simulink model "Langsdynamikmodell"  (R2021a)
settings: Solver=ode3  StartTime=0.0  StopTime=70  FixedStep=0.01  RelTol=1e-3
values from neighbouring files (symbols this model uses):
  A = 2    [Parameter.m]
  cw = 0.0    (= 0)    [Parameter.m]
  d = 0.63    [Parameter.m]
  m = 1500    [Parameter.m]
  p = 1.2    [Parameter.m]
undefined symbols (not defined in the file or in its folder): DiscIntNeverNeededParam
libraries: simulink x2
settings Model: Creator=ge78kon  LastModifiedBy=admin
settings SolverCC: AlgebraicLoopSolver=TrustRegion
settings DataIOCC: ReturnWorkspaceOutputs=off
settings DebuggingCC: SFMachineParentedDataDiag=warning  ArithmeticOperatorsInVariantConditions=warning
settings SFSimCC: CustomCodeUndefinedFunction=UseInterfaceOnly

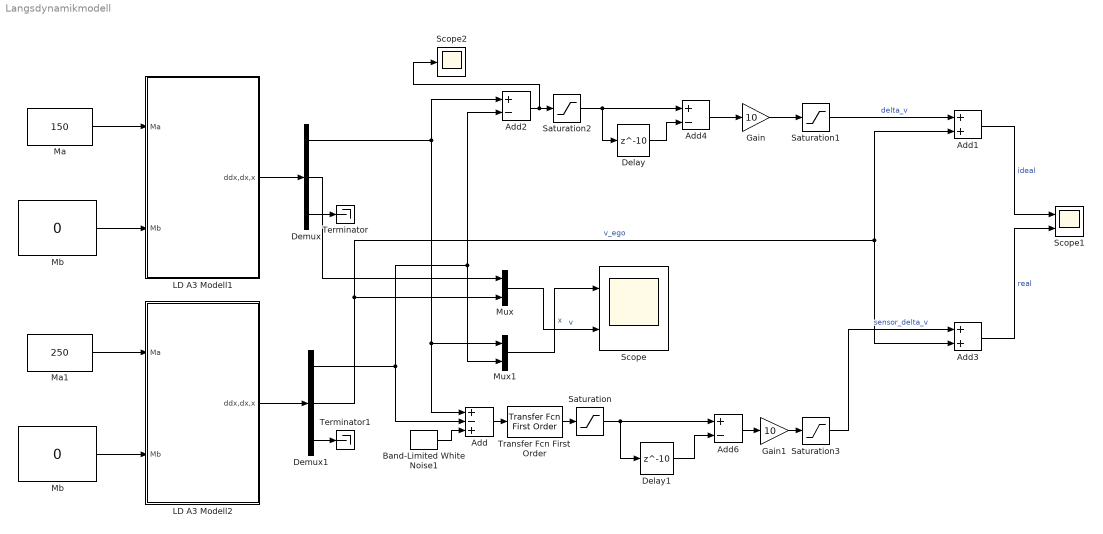
== system Langsdynamikmodell ==
  Add : Sum  Inputs=+-+
  Add1 : Sum
  Add2 : Sum  Inputs=+-
  Add3 : Sum
  Add4 : Sum  Inputs=+-
  Add6 : Sum  Inputs=+-
  Band-Limited White Noise1 : simulink/Sources/Band-Limited White Noise  Cov=[0.007]  Ts=0.01  seed=[23341]
  Delay : Delay  DelayLength=10
  Delay1 : Delay  DelayLength=10
  Demux : Demux  Outputs=3
  Demux1 : Demux  Outputs=3
  Gain : Gain  Gain=10
  Gain1 : Gain  Gain=10
  LD A3 Modell1 : Subsystem  mask{x_start=450, v_start=20}
      mask prompts: x_start "Startposition"; v_start "Startgeschwindigkeit"
  LD A3 Modell2 : Subsystem  mask{x_start=0, v_start=30}
      mask prompts: x_start "Startposition"; v_start "Startgeschwindigkeit"
  Ma : Constant  Value=150
  Ma1 : Constant  Value=250
  Mb : Constant  Value=0
  "Mb " : Constant  Value=0
  Mux : Mux  Inputs=2
  Mux1 : Mux  Inputs=2
  Saturation : Saturate  UpperLimit=200  LowerLimit=0
  Saturation1 : Saturate  UpperLimit=0  LowerLimit=-50
  Saturation2 : Saturate  UpperLimit=200  LowerLimit=0
  Saturation3 : Saturate  UpperLimit=0  LowerLimit=-50
  Scope : Scope  NumInputPorts=2
  Scope1 : Scope  NumInputPorts=2
  Scope2 : Scope
  Terminator : Terminator
  Terminator1 : Terminator
  Transfer Fcn First Order : simulink/Discrete/Transfer Fcn First Order  PoleZ=0.99  ICPrevOutput=0.0  DoSatur=off
  wires:
  Ma/1 -> LD A3 Modell1/1("Ma ")
  "Mb "/1 -> LD A3 Modell1/2("Mb ")
  LD A3 Modell1/1(ddx,dx,x) -> Demux/1
  LD A3 Modell2/1(ddx,dx,x) -> Demux1/1
  Ma1/1 -> LD A3 Modell2/1("Ma ")
  Mb/1 -> LD A3 Modell2/2("Mb ")
  Demux/3 -> Terminator/1
  Demux1/3 -> Terminator1/1
  Add6/1 -> Gain1/1
  Demux1/1 -> Add/2, Add2/2, Mux1/2
  Demux/2 -> Mux/1
  Demux1/2 -> Add1/2, Add3/2, Mux/2  "v_ego"
  Mux/1 -> Scope/2  "v"
  Mux1/1 -> Scope/1  "x"
  Add2/1 -> Scope2/1, Saturation2/1
  Add4/1 -> Gain/1
  Gain/1 -> Saturation1/1
  Band-Limited White Noise1/1 -> Add/3
  Demux/1 -> Mux1/1, Add/1, Add2/1
  Delay/1 -> Add4/2
  Delay1/1 -> Add6/2
  Saturation/1 -> Delay1/1, Add6/1
  Saturation2/1 -> Delay/1, Add4/1
  Saturation3/1 -> Add3/1  "sensor_delta_v"
  Add/1 -> Transfer Fcn First Order/1
  Gain1/1 -> Saturation3/1
  Transfer Fcn First Order/1 -> Saturation/1
  Saturation1/1 -> Add1/1  "delta_v"
  Add1/1 -> Scope1/1  "ideal"
  Add3/1 -> Scope1/2  "real"

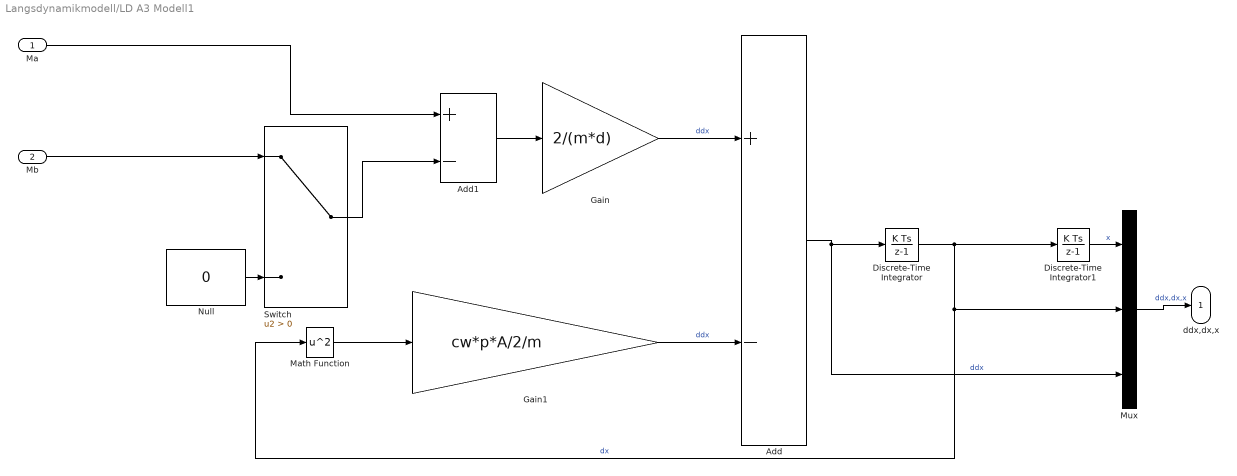
== system Langsdynamikmodell/LD A3 Modell1 ==
  "Ma " : Inport
  "Mb " : Inport  Port=2
  Add : Sum  Inputs=+-
  Add1 : Sum  Inputs=+-
  Discrete-Time Integrator : DiscreteIntegrator  InitialCondition=v_start  SampleTime=-1  ICPrevOutput=DiscIntNeverNeededParam  ICPrevScaledInput=DiscIntNeverNeededParam
  Discrete-Time Integrator1 : DiscreteIntegrator  InitialCondition=x_start  SampleTime=-1  ICPrevOutput=DiscIntNeverNeededParam  ICPrevScaledInput=DiscIntNeverNeededParam
  Gain : Gain  Gain=2/(m*d)
  Gain1 : Gain  Gain=cw*p*A/2/m
  Math Function : Math  Operator=square  SignedPower=on  SaturateOnIntegerOverflow=on
  Mux : Mux  Inputs=3
  Null : Constant  Value=0
  Switch : Switch  Criteria=u2 > Threshold
  ddx,dx,x : Outport  VectorParamsAs1DForOutWhenUnconnected=off
  wires:
  "Ma "/1 -> Add1/1
  Add1/1 -> Gain/1
  Discrete-Time Integrator/1 -> Math Function/1, Mux/2, Discrete-Time Integrator1/1  "dx"
  Gain1/1 -> Add/2  "ddx"
  Gain/1 -> Add/1  "ddx"
  Null/1 -> Switch/3
  Add/1 -> Discrete-Time Integrator/1, Mux/3  "ddx"
  Math Function/1 -> Gain1/1
  Switch/1 -> Add1/2
  Discrete-Time Integrator1/1 -> Mux/1  "x"
  "Mb "/1 -> Switch/1
  Mux/1 -> ddx,dx,x/1  "ddx,dx,x"

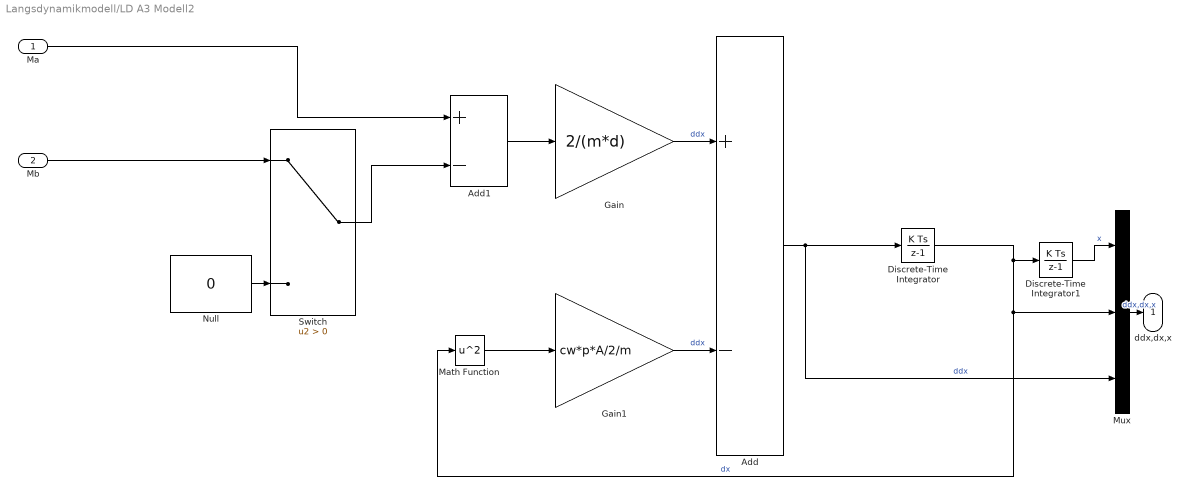
== system Langsdynamikmodell/LD A3 Modell2 ==
  "Ma " : Inport
  "Mb " : Inport  Port=2
  Add : Sum  Inputs=+-
  Add1 : Sum  Inputs=+-
  Discrete-Time Integrator : DiscreteIntegrator  InitialCondition=v_start  SampleTime=-1  ICPrevOutput=DiscIntNeverNeededParam  ICPrevScaledInput=DiscIntNeverNeededParam
  Discrete-Time Integrator1 : DiscreteIntegrator  InitialCondition=x_start  SampleTime=-1  ICPrevOutput=DiscIntNeverNeededParam  ICPrevScaledInput=DiscIntNeverNeededParam
  Gain : Gain  Gain=2/(m*d)
  Gain1 : Gain  Gain=cw*p*A/2/m
  Math Function : Math  Operator=square  SignedPower=on  SaturateOnIntegerOverflow=on
  Mux : Mux  Inputs=3
  Null : Constant  Value=0
  Switch : Switch  Criteria=u2 > Threshold
  ddx,dx,x : Outport  VectorParamsAs1DForOutWhenUnconnected=off
  wires:
  "Ma "/1 -> Add1/1
  Add1/1 -> Gain/1
  Discrete-Time Integrator/1 -> Mux/2, Math Function/1, Discrete-Time Integrator1/1  "dx"
  Gain1/1 -> Add/2  "ddx"
  Gain/1 -> Add/1  "ddx"
  Null/1 -> Switch/3
  Add/1 -> Discrete-Time Integrator/1, Mux/3  "ddx"
  Math Function/1 -> Gain1/1
  Switch/1 -> Add1/2
  Discrete-Time Integrator1/1 -> Mux/1  "x"
  "Mb "/1 -> Switch/1
  Mux/1 -> ddx,dx,x/1  "ddx,dx,x"
